simulink model "BEL073_6_STATCOM_MODELING"  (R2020a)
settings: Solver=VariableStepAuto  StartTime=0.0  StopTime=0.5  RelTol=1e-3
undefined symbols (not defined in the file): Cf, Lf, Lg, Rd, Rf, Rg
libraries: powerlib x16, powerlib_meascontrol x9, simulink x3
settings Model: Creator=Anil Lamichhane  LastModifiedBy=Anil Lamichhane

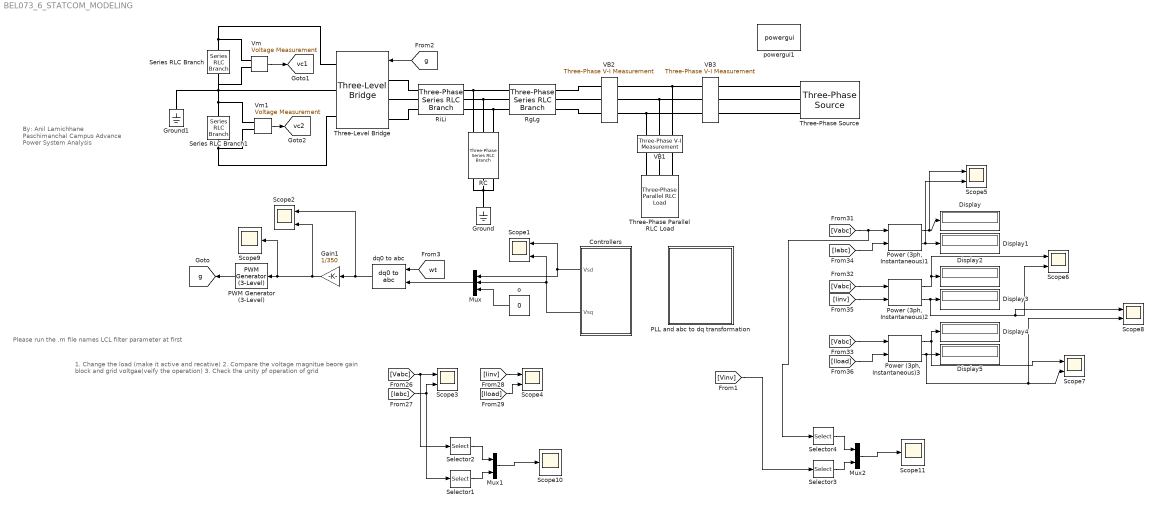
== system BEL073_6_STATCOM_MODELING ==
  note: Please run the .m file names LCL filter parameter at first
  note: By: Anil Lamichhane
      | Paschimanchal Campus
      | Advance Power System Analysis
  note: 1. Change the load (make it active and recative)
      | 2. Compare the voltage magnitue beore gain block and grid voltgae(veify the operation)
      | 3. Check the unity pf operation of grid
  Controllers : Subsystem
  Display{,1..5} (6 alike) : Display
  Gain1 : Gain  Gain=1/350
  Ground : powerlib/Elements/Ground  LConnTagsString=a
  Ground1 : powerlib/Elements/Ground  LConnTagsString=a
  Mux : Mux  Inputs=3
  Mux1 : Mux  Inputs=2
  Mux2 : Mux  Inputs=2
  "PLL and abc to dq transformation " : Subsystem
  PWM Generator (3-Level) : powerlib_meascontrol/Pulse & Signal Generators/PWM Generator (3-Level)  ModulatorType=Three-phase bridge (12 pulses)  ModulatorMode=Unsynchronized  nF=27  Fc=10000  ModulatingSignals=off  m=0.8  Freq=60  Phase=0  Ts=0
      settings: SourceProductBaseCode=PS
  "Power (3ph, Instantaneous)1" : powerlib_meascontrol/Measurements/Power (3ph, Instantaneous)
  "Power (3ph, Instantaneous)2" : powerlib_meascontrol/Measurements/Power (3ph, Instantaneous)
  "Power (3ph, Instantaneous)3" : powerlib_meascontrol/Measurements/Power (3ph, Instantaneous)
  RC : powerlib/Elements/Three-Phase Series RLC Branch  LConnTagsString=A|B|C  RConnTagsString=A|B|C  BranchType=RC  Resistance=Rd  Inductance=1e-3  Capacitance=Cf  Measurements=None
  RgLg : powerlib/Elements/Three-Phase Series RLC Branch  LConnTagsString=A|B|C  RConnTagsString=A|B|C  BranchType=RL  Resistance=Rg  Inductance=Lg  Capacitance=1e-6  Measurements=None
  RiLi : powerlib/Elements/Three-Phase Series RLC Branch  LConnTagsString=A|B|C  RConnTagsString=A|B|C  BranchType=RL  Resistance=Rf  Inductance=Lf  Capacitance=1e-6  Measurements=None
  Scope{1..8} (8 alike) : Scope  NumInputPorts=2
  Scope10 : Scope
  Scope11 : Scope
  Scope9 : Scope
  Selector{1..4} (4 alike) : Selector  InputPortWidth=3  IndexOptions=Index vector (dialog)  Indices=[1 ]  OutputSizes=1
  Series RLC Branch : powerlib/Elements/Series RLC Branch  LConnTagsString=__new0  RConnTagsString=__new0  BranchType=C  Resistance=1  Inductance=1e-3  SetiL0=off  InitialCurrent=0  Capacitance=46000e-6  Setx0=on  InitialVoltage=350  Measurements=None
  Series RLC Branch1 : powerlib/Elements/Series RLC Branch  LConnTagsString=__new0  RConnTagsString=__new0  BranchType=C  Resistance=1  Inductance=1e-3  SetiL0=off  InitialCurrent=0  Capacitance=46000e-6  Setx0=on  InitialVoltage=350  Measurements=None
  Three-Level Bridge : powerlib/Power Electronics/Three-Level Bridge  Arms=3  SnubberResistance=1e5  SbubberCapacitance=inf  Device=IGBT / Diodes  Ron=1e-3  ForwardVoltages="[  0  0  ]"  Measurements=None
      settings: SourceProductBaseCode=PS
  Three-Phase Parallel RLC Load : powerlib/Elements/Three-Phase Parallel RLC Load  LConnTagsString=A|B|C  Configuration=Y (grounded)  NominalVoltage=380  Vabc=[1e3 1e3 1e3]  Vabcp=[1e3 1e3 1e3]  NominalFrequency=50  UnbalancedPower=off  ActivePower=3e3  InductivePower=0  CapacitivePower=5e3  Pabc=[10e3 9e3 11e3]  QLabc=[100 90 110]  QCabc=[100 90 110]  Pabcp=[10e3 9e3 11e3]  QLabcp=[100 90 110]  QCabcp=[100 90 110]  Measurements=None  LoadType=constant Z
  Three-Phase Source : powerlib/Electrical Sources/Three-Phase Source  InternalConnection=Yg  VoltagePhases=off  Voltage=380  PhaseAngle=0  Voltage_phases=[25e3 25e3 25e3]/sqrt(3)  PhaseAngles_phases=[0 -120 +120]  Frequency=50  NonIdealSource=on  SpecifyImpedance=off  Resistance=0.08929  Inductance=16.58e-6  ShortCircuitLevel=100e6  BaseVoltage=380  XRratio=7  BusType=swing  Pref=10e3  Qref=0  Prefabc=[10e3, 10e3, 10e3]  Qrefabc=[0, 0, 0]  Qmin=-inf  Qmax=inf
  VB1 : powerlib/Measurements/Three-Phase V-I Measurement  VoltageMeasurement=phase-to-ground  SetLabelV=on  LabelV=Vload  Vpu=off  VpuLL=off  CurrentMeasurement=yes  SetLabelI=on  LabelI=Iload  Ipu=off  Pbase=100e6  Vbase=500e3  OutputType=Complex  PhasorSimulation=off  PSBequivalent=0
  VB2 : powerlib/Measurements/Three-Phase V-I Measurement  VoltageMeasurement=phase-to-ground  SetLabelV=on  LabelV=Vinv  Vpu=off  VpuLL=off  CurrentMeasurement=yes  SetLabelI=on  LabelI=Iinv  Ipu=off  Pbase=100e6  Vbase=500e3  OutputType=Complex  PhasorSimulation=off  PSBequivalent=0
  VB3 : powerlib/Measurements/Three-Phase V-I Measurement  VoltageMeasurement=phase-to-ground  SetLabelV=on  LabelV=Vabc  Vpu=off  VpuLL=off  CurrentMeasurement=yes  SetLabelI=on  LabelI=Iabc  Ipu=off  Pbase=100e6  Vbase=500e3  OutputType=Complex  PhasorSimulation=off  PSBequivalent=0
  Vm : powerlib/Measurements/Voltage Measurement  PhasorSimulation=off  OutputType=Complex  PSBequivalent=0
  Vm1 : powerlib/Measurements/Voltage Measurement  PhasorSimulation=off  OutputType=Complex  PSBequivalent=0
  dq0 to abc : powerlib_meascontrol/Transformations/dq0 to abc  Alignment=90 degrees behind phase A axis
  o : Constant  Value=0
  powergui1 : powerlib/powergui  Priority=1  SimulationMode=Continuous  SampleTime=1e-6  frequency=60  Iterations=50  frequencyindice=50  Pbase=100e6  ErrMax=1e-4  UnitsV=kV  UnitsW=MW  buscounter=0  FunctionMessages=off  echomessages=off  EnableUseOfTLC=off  CurrentSourceSwitches=off  DisableSnubberDevices=off  DisableRonSwitches=off  DisableVfSwitches=off  DisplayEquations=off  AutomaticDiscreteSolvers=off  SolverType=Tustin/Backward Euler (TBE)  Interpol=off  ExternalGateDelay=off  methode=off  Ts=100  x0status=blocks  SPID=on  SwTol=0  HookPort=off  NonlinearTolerance=1e-4  nMaxIteration=100  ContinueOnMaxIteration=off  RestoreLinks=warning  ResistiveCurrentMeasurement=off  Frange=[0:2:500]  Ylog=off  Xlog=on  ShowGrid=off  save=off  variable=ZData  structure=grid  ZoomFFT=off  StartTime=0.2  cycles=1  DisplayStyle=1  fundamental=50  FreqAxis=off  MaxFrequency=800  frequencyindicesteady=1  RmsSteady=1  display=off
  tag scope: g=global, vc1=global, vc2=global
  wires:
  Vm1/1 -> [vc2]
  Vm/1 -> [vc1]
  Gain1/1 -> Scope9/1, PWM Generator (3-Level)/1, Scope2/2
  Controllers/2(Vsq) -> Mux/2, Scope1/2
  Controllers/1(Vsd) -> Scope1/1, Mux/1
  o/1 -> Mux/3
  dq0 to abc/1 -> Scope2/1, Gain1/1
  Mux/1 -> dq0 to abc/1
  [g] -> Three-Level Bridge/1
  [wt] -> dq0 to abc/2
  PWM Generator (3-Level)/1 -> [g]
  [Iinv] -> Scope4/1
  [Iload] -> Scope4/2
  [Iload] -> "Power (3ph, Instantaneous)3"/2
  [Iabc] -> "Power (3ph, Instantaneous)1"/2
  [Iinv] -> "Power (3ph, Instantaneous)2"/2
  [Vabc] -> "Power (3ph, Instantaneous)2"/1
  [Vabc] -> "Power (3ph, Instantaneous)3"/1
  "Power (3ph, Instantaneous)2"/2 -> Scope8/1, Scope6/2, Display3/1
  "Power (3ph, Instantaneous)3"/2 -> Scope8/2, Scope7/2, Display5/1
  "Power (3ph, Instantaneous)2"/1 -> Scope6/1, Display2/1
  "Power (3ph, Instantaneous)1"/2 -> Display1/1, Scope5/2
  "Power (3ph, Instantaneous)1"/1 -> Scope5/1, Display/1
  "Power (3ph, Instantaneous)3"/1 -> Display4/1, Scope7/1
  Selector1/1 -> Mux1/2
  [Vabc] -> Selector2/1, Scope3/1
  [Iabc] -> Scope3/2, Selector1/1
  Selector2/1 -> Mux1/1
  Mux1/1 -> Scope10/1
  Mux2/1 -> Scope11/1
  [Vinv] -> Selector3/1
  Selector4/1 -> Mux2/1
  [Vabc] -> Selector4/1, "Power (3ph, Instantaneous)1"/1
  Selector3/1 -> Mux2/2
  connections:
  RiLi/RConn1 -- RgLg/LConn1 -- RC/LConn1
  Vm1/LConn2 -- Three-Level Bridge/RConn3 -- Series RLC Branch1/RConn1
  VB1/LConn1 -- VB3/RConn1 -- VB2/RConn1
  RgLg/LConn2 -- RiLi/RConn2 -- RC/LConn2
  Vm1/LConn1 -- Ground1/LConn1 -- Vm/LConn2 -- Series RLC Branch/RConn1 -- Three-Level Bridge/RConn2 -- Series RLC Branch1/LConn1
  VB1/LConn3 -- VB3/RConn3 -- VB2/RConn3
  RC/RConn1 -- Ground/LConn1 -- RC/RConn2 -- RC/RConn3
  Series RLC Branch/LConn1 -- Three-Level Bridge/RConn1 -- Vm/LConn1
  RC/LConn3 -- RiLi/RConn3 -- RgLg/LConn3
  VB1/LConn2 -- VB3/RConn2 -- VB2/RConn2
  Three-Level Bridge/LConn1 -- RiLi/LConn1
  VB3/LConn1 -- Three-Phase Source/RConn1
  VB3/LConn2 -- Three-Phase Source/RConn2
  VB3/LConn3 -- Three-Phase Source/RConn3
  Three-Level Bridge/LConn2 -- RiLi/LConn2
  Three-Level Bridge/LConn3 -- RiLi/LConn3
  VB1/RConn3 -- Three-Phase Parallel RLC Load/LConn1
  VB1/RConn2 -- Three-Phase Parallel RLC Load/LConn2
  VB1/RConn1 -- Three-Phase Parallel RLC Load/LConn3
  VB2/LConn1 -- RgLg/RConn1
  RgLg/RConn2 -- VB2/LConn2
  RgLg/RConn3 -- VB2/LConn3

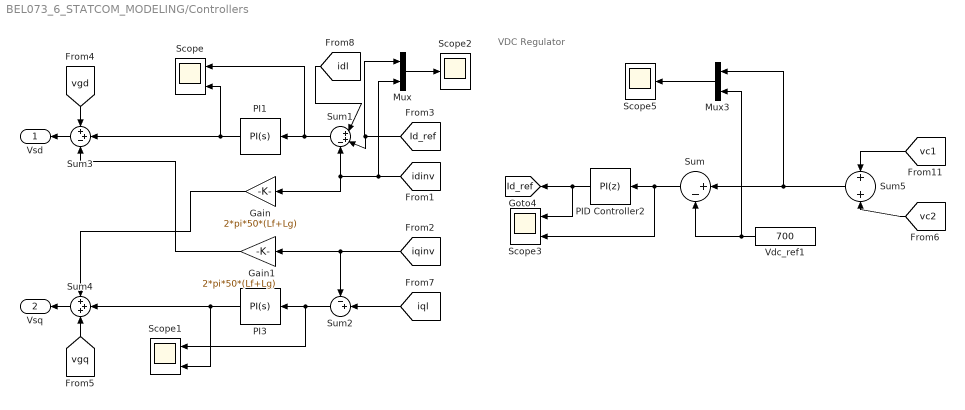
== system BEL073_6_STATCOM_MODELING/Controllers ==
  note: VDC Regulator
  Gain : Gain  Gain=2*pi*50*(Lf+Lg)
  Gain1 : Gain  Gain=2*pi*50*(Lf+Lg)
  Mux : Mux  Inputs=2
  Mux3 : Mux  Inputs=2
  PI1 : simulink/Continuous/PID Controller  Controller=PI  Form=Parallel  TimeDomain=Continuous-time  UseExternalTs=off  SampleTime=-1  IntegratorMethod=Forward Euler  FilterMethod=Forward Euler  ControllerParametersSource=internal  P=1.45  I=137  D=0  UseFilter=on  N=100  TunerSelectOption=Transfer Function Based (PID Tuner App)  InitialConditionSource=internal  InitialConditionForIntegrator=0  InitialConditionForFilter=0  DifferentiatorICPrevScaledInput=0  ExternalReset=none  TrackingMode=off  Kt=1  LimitOutput=off  UpperSaturationLimit=inf  LowerSaturationLimit=-inf  LinearizeAsGain=on  AntiWindupMode=none  Kb=1  POutMin=[]  POutMax=[]  IOutMin=[]  IOutMax=[]  DOutMin=[]  DOutMax=[]  NOutMin=[]  NOutMax=[]  SumOutMin=[]  SumOutMax=[]  SaturationOutMin=[]  SaturationOutMax=[]  PParamMin=[]  PParamMax=[]  IParamMin=[]  IParamMax=[]  DParamMin=[]  DParamMax=[]  NParamMin=[]  NParamMax=[]  KbParamMin=[]  KbParamMax=[]  KtParamMin=[]  KtParamMax=[]  KbOutMin=[]  KbOutMax=[]  KtOutMin=[]  KtOutMax=[]  IntegratorOutMin=[]  IntegratorOutMax=[]  FilterOutMin=[]  FilterOutMax=[]  SumI1OutMin=[]  SumI1OutMax=[]  SumI2OutMin=[]  SumI2OutMax=[]  SumI3OutMin=[]  SumI3OutMax=[]  SumI4OutMin=[]  SumI4OutMax=[]  SumDOutMin=[]  SumDOutMax=[]  DifferentiatorOutMin=[]  DifferentiatorOutMax=[]  FilterDiffOutCoefMin=[]  FilterDiffOutCoefMax=[]  ReciprocalOutMin=[]  ReciprocalOutMax=[]  SumDenOutMin=[]  SumDenOutMax=[]  SumNumOutMin=[]  SumNumOutMax=[]  DivideOutMin=[]  DivideOutMax=[]  UdiffTsProdOutMin=[]  UdiffTsProdOutMax=[]  NTsProdOutMin=[]  NTsProdOutMax=[]  UintegralTsProdOutMin=[]  UintegralTsProdOutMax=[]  UngainTsProdOutMin=[]  UngainTsProdOutMax=[]  IntegratorContinuousStateAttributes=''  IntegratorStateMustResolveToSignalObject=off  IntegratorRTWStateStorageClass=Auto  FilterContinuousStateAttributes=''  FilterStateMustResolveToSignalObject=off  FilterRTWStateStorageClass=Auto  ParallelPVariant=InternalParameters  IdealPVariant=Disabled  IVariant=InternalParameters  DVariant=Disabled  IntegratorVariant=Continuous  SatVariant=Disabled  AWVariant=Passthrough  PCopyVariant=Disabled  TRVariant=Disabled  FdbkBlocksVariant=Forward  IdealPFdbkVariant=Disabled  SatFdbkVariant=Disabled  DerivativeFilterVariant=Disabled  NVariant=Disabled  NCopyVariant=Disabled_SignalSpec  FilterICVariant=Disabled  IntegratorICVariant=InternalICs  ExternalResetVariant=Disabled  TRSumVariant=Passthrough  SumFdbkVariant=Disabled  SumVariant=Sum_PI  TsampFilterVariant=InternalTs  TsampNgainVariant=Passthrough  TsampIntegralVariant=Passthrough
  PI3 : simulink/Continuous/PID Controller  Controller=PI  Form=Parallel  TimeDomain=Continuous-time  UseExternalTs=off  SampleTime=-1  IntegratorMethod=Forward Euler  FilterMethod=Forward Euler  ControllerParametersSource=internal  P=1.45  I=137  D=0  UseFilter=on  N=100  TunerSelectOption=Transfer Function Based (PID Tuner App)  InitialConditionSource=internal  InitialConditionForIntegrator=0  InitialConditionForFilter=0  DifferentiatorICPrevScaledInput=0  ExternalReset=none  TrackingMode=off  Kt=1  LimitOutput=off  UpperSaturationLimit=inf  LowerSaturationLimit=-inf  LinearizeAsGain=on  AntiWindupMode=none  Kb=1  POutMin=[]  POutMax=[]  IOutMin=[]  IOutMax=[]  DOutMin=[]  DOutMax=[]  NOutMin=[]  NOutMax=[]  SumOutMin=[]  SumOutMax=[]  SaturationOutMin=[]  SaturationOutMax=[]  PParamMin=[]  PParamMax=[]  IParamMin=[]  IParamMax=[]  DParamMin=[]  DParamMax=[]  NParamMin=[]  NParamMax=[]  KbParamMin=[]  KbParamMax=[]  KtParamMin=[]  KtParamMax=[]  KbOutMin=[]  KbOutMax=[]  KtOutMin=[]  KtOutMax=[]  IntegratorOutMin=[]  IntegratorOutMax=[]  FilterOutMin=[]  FilterOutMax=[]  SumI1OutMin=[]  SumI1OutMax=[]  SumI2OutMin=[]  SumI2OutMax=[]  SumI3OutMin=[]  SumI3OutMax=[]  SumI4OutMin=[]  SumI4OutMax=[]  SumDOutMin=[]  SumDOutMax=[]  DifferentiatorOutMin=[]  DifferentiatorOutMax=[]  FilterDiffOutCoefMin=[]  FilterDiffOutCoefMax=[]  ReciprocalOutMin=[]  ReciprocalOutMax=[]  SumDenOutMin=[]  SumDenOutMax=[]  SumNumOutMin=[]  SumNumOutMax=[]  DivideOutMin=[]  DivideOutMax=[]  UdiffTsProdOutMin=[]  UdiffTsProdOutMax=[]  NTsProdOutMin=[]  NTsProdOutMax=[]  UintegralTsProdOutMin=[]  UintegralTsProdOutMax=[]  UngainTsProdOutMin=[]  UngainTsProdOutMax=[]  IntegratorContinuousStateAttributes=''  IntegratorStateMustResolveToSignalObject=off  IntegratorRTWStateStorageClass=Auto  FilterContinuousStateAttributes=''  FilterStateMustResolveToSignalObject=off  FilterRTWStateStorageClass=Auto  ParallelPVariant=InternalParameters  IdealPVariant=Disabled  IVariant=InternalParameters  DVariant=Disabled  IntegratorVariant=Continuous  SatVariant=Disabled  AWVariant=Passthrough  PCopyVariant=Disabled  TRVariant=Disabled  FdbkBlocksVariant=Forward  IdealPFdbkVariant=Disabled  SatFdbkVariant=Disabled  DerivativeFilterVariant=Disabled  NVariant=Disabled  NCopyVariant=Disabled_SignalSpec  FilterICVariant=Disabled  IntegratorICVariant=InternalICs  ExternalResetVariant=Disabled  TRSumVariant=Passthrough  SumFdbkVariant=Disabled  SumVariant=Sum_PI  TsampFilterVariant=InternalTs  TsampNgainVariant=Passthrough  TsampIntegralVariant=Passthrough
  PID Controller2 : simulink/Continuous/PID Controller  Controller=PI  Form=Ideal  TimeDomain=Discrete-time  UseExternalTs=off  SampleTime=-1  IntegratorMethod=Forward Euler  FilterMethod=Forward Euler  ControllerParametersSource=internal  P=1.61  I=123  D=1  UseFilter=on  N=26964.3518480036  TunerSelectOption=Transfer Function Based (PID Tuner App)  InitialConditionSource=internal  InitialConditionForIntegrator=0  InitialConditionForFilter=0  DifferentiatorICPrevScaledInput=0  ExternalReset=none  TrackingMode=off  Kt=1  LimitOutput=off  UpperSaturationLimit=inf  LowerSaturationLimit=-inf  LinearizeAsGain=on  AntiWindupMode=none  Kb=1  POutMin=[]  POutMax=[]  IOutMin=[]  IOutMax=[]  DOutMin=[]  DOutMax=[]  NOutMin=[]  NOutMax=[]  SumOutMin=[]  SumOutMax=[]  SaturationOutMin=[]  SaturationOutMax=[]  PParamMin=[]  PParamMax=[]  IParamMin=[]  IParamMax=[]  DParamMin=[]  DParamMax=[]  NParamMin=[]  NParamMax=[]  KbParamMin=[]  KbParamMax=[]  KtParamMin=[]  KtParamMax=[]  KbOutMin=[]  KbOutMax=[]  KtOutMin=[]  KtOutMax=[]  IntegratorOutMin=[]  IntegratorOutMax=[]  FilterOutMin=[]  FilterOutMax=[]  SumI1OutMin=[]  SumI1OutMax=[]  SumI2OutMin=[]  SumI2OutMax=[]  SumI3OutMin=[]  SumI3OutMax=[]  SumI4OutMin=[]  SumI4OutMax=[]  SumDOutMin=[]  SumDOutMax=[]  DifferentiatorOutMin=[]  DifferentiatorOutMax=[]  FilterDiffOutCoefMin=[]  FilterDiffOutCoefMax=[]  ReciprocalOutMin=[]  ReciprocalOutMax=[]  SumDenOutMin=[]  SumDenOutMax=[]  SumNumOutMin=[]  SumNumOutMax=[]  DivideOutMin=[]  DivideOutMax=[]  UdiffTsProdOutMin=[]  UdiffTsProdOutMax=[]  NTsProdOutMin=[]  NTsProdOutMax=[]  UintegralTsProdOutMin=[]  UintegralTsProdOutMax=[]  UngainTsProdOutMin=[]  UngainTsProdOutMax=[]  IntegratorContinuousStateAttributes=''  IntegratorStateMustResolveToSignalObject=off  IntegratorRTWStateStorageClass=Auto  FilterContinuousStateAttributes=''  FilterStateMustResolveToSignalObject=off  FilterRTWStateStorageClass=Auto  ParallelPVariant=Passthrough  IdealPVariant=InternalParameters  IVariant=InternalParameters  DVariant=Disabled  IntegratorVariant=Discrete  SatVariant=Disabled  AWVariant=Passthrough  PCopyVariant=Disabled  TRVariant=Disabled  FdbkBlocksVariant=Forward  IdealPFdbkVariant=Disabled  SatFdbkVariant=Disabled  DerivativeFilterVariant=Disabled  NVariant=Disabled  NCopyVariant=Disabled_SignalSpec  FilterICVariant=Disabled  IntegratorICVariant=InternalICs  ExternalResetVariant=Disabled  TRSumVariant=Passthrough  SumFdbkVariant=Disabled  SumVariant=Sum_PI  TsampFilterVariant=InternalTs  TsampNgainVariant=Passthrough  TsampIntegralVariant=Passthrough
  Scope : Scope  NumInputPorts=2
  Scope1 : Scope  NumInputPorts=2
  Scope2 : Scope
  Scope3 : Scope  NumInputPorts=2
  Scope5 : Scope
  Sum : Sum  Inputs=|+-
  Sum1 : Sum  Inputs=|++-
  Sum2 : Sum  Inputs=-+|
  Sum3 : Sum  Inputs=++-
  Sum4 : Sum  Inputs=+++
  Sum5 : Sum
  Vdc_ref1 : Constant  Value=700
  Vsd : Outport
  Vsq : Outport  Port=2
  tag scope: Id_ref=global
  wires:
  [vgq] -> Sum4/3
  Gain/1 -> Sum4/1
  [iqinv] -> Sum2/1, Gain1/1
  Gain1/1 -> Sum3/3
  [idinv] -> Mux/2, Gain/1, Sum1/3
  Sum2/1 -> PI3/1, Scope1/1
  [vgd] -> Sum3/1
  Sum1/1 -> Scope/1, PI1/1
  Sum4/1 -> Vsq/1
  Sum3/1 -> Vsd/1
  [iql] -> Sum2/2
  PI3/1 -> Scope1/2, Sum4/2
  PI1/1 -> Scope/2, Sum3/2
  Mux/1 -> Scope2/1
  [Id_ref] -> Sum1/2, Mux/1
  Mux3/1 -> Scope5/1
  Sum5/1 -> Mux3/1, Sum/1
  [vc2] -> Sum5/2
  [vc1] -> Sum5/1
  Sum/1 -> Scope3/2, PID Controller2/1
  PID Controller2/1 -> Scope3/1, [Id_ref]
  Vdc_ref1/1 -> Mux3/2, Sum/2
  [idl] -> Sum1/1

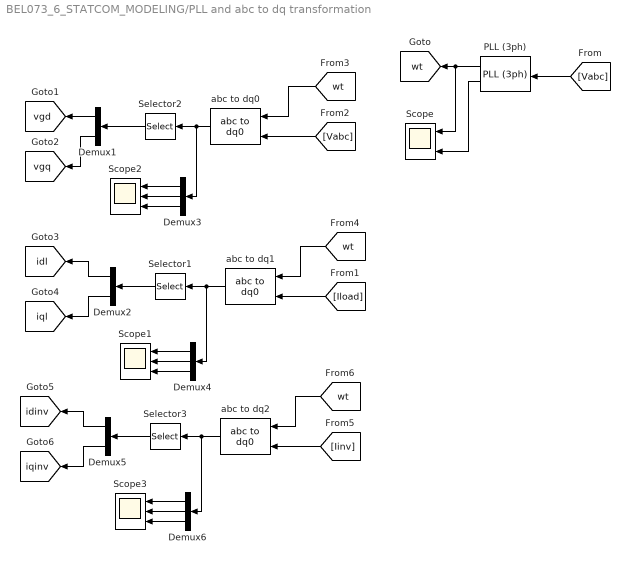
== system BEL073_6_STATCOM_MODELING/PLL and abc to dq transformation  ==
  Demux1 : Demux  Outputs=2
  Demux2 : Demux  Outputs=2
  Demux3 : Demux  Outputs=3
  Demux4 : Demux  Outputs=3
  Demux5 : Demux  Outputs=2
  Demux6 : Demux  Outputs=3
  PLL (3ph) : powerlib_meascontrol/PLL/PLL (3ph)  Fmin=45  Par_Init=[0, 50]  ParK=[180, 3200, 1]  TcD=1e-4  MaxRateChangeFreq=12  FilterCutOffFreq=25  Ts=0  AGC=on
  Scope : Scope  NumInputPorts=2
  Scope1 : Scope  NumInputPorts=3
  Scope2 : Scope  NumInputPorts=3
  Scope3 : Scope  NumInputPorts=3
  Selector1 : Selector  InputPortWidth=3  IndexOptions=Index vector (dialog)  Indices=[1 2]  OutputSizes=1
  Selector2 : Selector  InputPortWidth=3  IndexOptions=Index vector (dialog)  Indices=[1 2]  OutputSizes=1
  Selector3 : Selector  InputPortWidth=3  IndexOptions=Index vector (dialog)  Indices=[1 2]  OutputSizes=1
  abc to dq0 : powerlib_meascontrol/Transformations/abc to dq0  Alignment=90 degrees behind phase A axis
  abc to dq1 : powerlib_meascontrol/Transformations/abc to dq0  Alignment=90 degrees behind phase A axis
  abc to dq2 : powerlib_meascontrol/Transformations/abc to dq0  Alignment=90 degrees behind phase A axis
  tag scope: idinv=global, idl=global, iqinv=global, iql=global, vgd=global, vgq=global, wt=global
  wires:
  PLL (3ph)/1 -> Scope/2
  [Vabc] -> abc to dq0/1
  abc to dq0/1 -> Demux3/1, Selector2/1
  [wt] -> abc to dq1/2
  [wt] -> abc to dq0/2
  [Iload] -> abc to dq1/1
  [Vabc] -> PLL (3ph)/1
  PLL (3ph)/2 -> Scope/1, [wt]
  Demux1/2 -> [vgq]
  Demux2/1 -> [idl]
  Demux2/2 -> [iql]
  Demux1/1 -> [vgd]
  Selector1/1 -> Demux2/1
  Selector2/1 -> Demux1/1
  Demux3/1 -> Scope2/1
  Demux3/2 -> Scope2/2
  Demux3/3 -> Scope2/3
  Demux4/3 -> Scope1/3
  Demux4/1 -> Scope1/1
  abc to dq1/1 -> Demux4/1, Selector1/1
  Demux4/2 -> Scope1/2
  Demux6/3 -> Scope3/3
  Demux6/1 -> Scope3/1
  Demux5/2 -> [iqinv]
  Demux5/1 -> [idinv]
  [Iinv] -> abc to dq2/1
  Selector3/1 -> Demux5/1
  abc to dq2/1 -> Demux6/1, Selector3/1
  [wt] -> abc to dq2/2
  Demux6/2 -> Scope3/2
